simulink model "MRA"  (R2020b)
settings: Solver=VariableStepAuto  StartTime=0.0  StopTime=tsim  MaxStep=0.01  RelTol=1e-3
values from neighbouring files (symbols this model uses):
  c = 10    [SistemaMasaResorteAmortiguador.m]
  F = 1    [SistemaMasaResorteAmortiguador.m]
  k = 20    [SistemaMasaResorteAmortiguador.m]
  m = 2    [SistemaMasaResorteAmortiguador.m]
settings Model: Creator=Sergio  LastModifiedBy=cesar
settings DataIOCC: ReturnWorkspaceOutputs=off
settings DebuggingCC: ArithmeticOperatorsInVariantConditions=warning
settings SFSimCC: SimUseLocalCustomCode=off  CustomCodeUndefinedFunction=UseInterfaceOnly
settings RTWCC: RTWUseLocalCustomCode=off

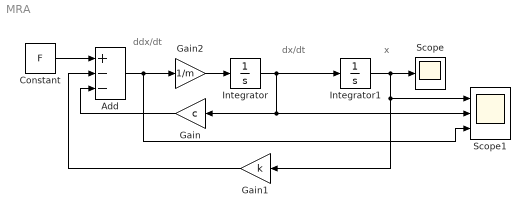
== system MRA ==
  note: ddx/dt
  note: dx/dt
  note: x
  Add : Sum  Inputs=+--
  Constant : Constant  Value=F
  Gain : Gain  Gain=c
  Gain1 : Gain  Gain=k
  Gain2 : Gain  Gain=1/m
  Integrator : Integrator
  Integrator1 : Integrator
  Scope : Scope
  Scope1 : Scope  NumInputPorts=3
  wires:
  Gain2/1 -> Integrator/1
  Integrator/1 -> Integrator1/1, Scope1/2, Gain/1
  Constant/1 -> Add/1
  Gain/1 -> Add/3
  Integrator1/1 -> Scope/1, Gain1/1, Scope1/1
  Gain1/1 -> Add/2
  Add/1 -> Scope1/3, Gain2/1
